simulink model "verify_SumTime_mdl"  (R2016b)
settings: Solver=VariableStepAuto  StartTime=0  StopTime=24*3600+1  MaxStep=1800  RelTol=1e-3  EnableMultiTasking=on
libraries: carnot x2
settings Model: Creator=drhf  LastModifiedBy=drhf
settings DataIOCC: SaveFormat=Array  SignalLoggingSaveFormat=ModelDataLogs
settings OptimizationCC: ExpressionDepthLimit=2147483647  LifeSpan=inf
settings DebuggingCC: UnderspecifiedInitializationDetection=Classic  MergeDetectMultiDrivingBlocksExec=none  SolverPrmCheckMsg=warning  FcnCallInpInsideContextMsg=warning  StateNameClashWarn=warning  SFUnexpectedBacktrackingDiag=warning  SFNoUnconditionalDefaultTransitionDiag=warning  SFExecutionAtInitializationDiag=none
settings HardwareCC: ProdBitPerPointer=32  ProdBitPerSizeT=32  ProdBitPerPtrDiffT=32  ProdLargestAtomicFloat=None  ProdIntDivRoundTo=Undefined  ProdEndianess=Unspecified  ProdWordSize=32  ProdHWDeviceType=32-bit Generic
settings ModelReferenceCC: PropagateSignalLabelsOutOfModel=off
settings GRTTargetCC: TargetLangStandard=C89/C90 (ANSI)  GeneratePreprocessorConditionals=Disable all  CombineOutputUpdateFcns=off  GRTInterface=on
settings ConfigComp: CovMetricSettings=dw  CovHtmlReporting=on  CovSaveCumulativeToWorkspaceVar=on  CovSaveSingleToWorkspaceVar=on  CovExternalEMLEnable=off

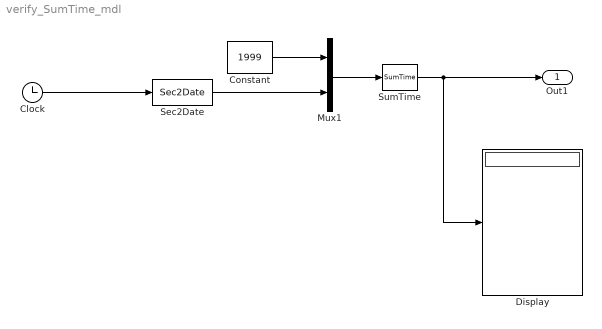
== system verify_SumTime_mdl ==
  Clock : Clock
  Constant : Constant  Value=1999
  Display : Display
  Mux1 : Mux  Inputs=2
  Sec2Date : carnot/Toolbox/Sec2Date
  SumTime : carnot/Toolbox/SumTime
  Out1 : Outport
  wires:
  SumTime/1 -> Display/1, Out1/1
  Sec2Date/1 -> Mux1/2
  Clock/1 -> Sec2Date/1
  Mux1/1 -> SumTime/1
  Constant/1 -> Mux1/1
